simulink model "SimpleEKF_2007a"  (Simulink 6.6)
settings: Solver=FixedStepDiscrete  StartTime=0.0  StopTime=300  FixedStep=0.01  RelTol=1e-3
values from neighbouring files (symbols this model uses):
  initP = diag([ 1 1 1 1e5 1e5 1 1e5 1e5 1e5 ])    [SimpleEKF_init.m.m]
undefined symbols (not defined in the file or in its folder): DiscIntNeverNeededParam, gcbh, hwbcalib_subsystem
libraries: simulink x8, dspmtrx3 x5, dspinverses x1
(part 7 of 9)

== system SimpleEKF_2007a/INS/Attitude update/Stage1/Subsystem1/a4 ==
  attInitCon : Inport  OutDataType=fixdt(1,16,0)  OutScaling=[]
  Demux : Demux  Outputs=3
  Gain : Gain  Gain=0.5  ParameterDataType=fixdt(1,16,0)  ParameterScaling=[]  OutDataType=fixdt(1,16,0)  OutScaling=[]  SampleTime=0.01
  Gain1 : Gain  Gain=0.5  ParameterDataType=fixdt(1,16,0)  ParameterScaling=[]  OutDataType=fixdt(1,16,0)  OutScaling=[]  SampleTime=0.01
  Gain2 : Gain  Gain=0.5  ParameterDataType=fixdt(1,16,0)  ParameterScaling=[]  OutDataType=fixdt(1,16,0)  OutScaling=[]  SampleTime=0.01
  Product : Product  Inputs=3  OutDataType=fixdt(1,16,0)  OutScaling=[]  SampleTime=0.01  RndMeth=Zero
  Product1 : Product  Inputs=3  OutDataType=fixdt(1,16,0)  OutScaling=[]  SampleTime=0.01  RndMeth=Zero
  Sum : Sum  Inputs=|+-  OutDataType=fixdt(1,16,0)  OutScaling=[]  SampleTime=0.01
  Trigonometric Function : Trigonometry  Operator=cos  SampleTime=0.01
  Trigonometric Function1 : Trigonometry  Operator=cos  SampleTime=0.01
  Trigonometric Function2 : Trigonometry  SampleTime=0.01
  Trigonometric Function3 : Trigonometry
  Trigonometric Function4 : Trigonometry  Operator=cos  SampleTime=0.01
  Trigonometric Function5 : Trigonometry  SampleTime=0.01
  a2 : Outport  OutDataType=fixdt(1,16,0)  OutScaling=[]
  wires:
  attInitCon/1 -> Demux/1
  Demux/1 -> Gain2/1
  Demux/2 -> Gain/1
  Demux/3 -> Gain1/1
  Gain2/1 -> Trigonometric Function/1, Trigonometric Function3/1
  Gain/1 -> Trigonometric Function1/1, Trigonometric Function5/1
  Gain1/1 -> Trigonometric Function2/1, Trigonometric Function4/1
  Trigonometric Function/1 -> Product/1
  Trigonometric Function1/1 -> Product/2
  Trigonometric Function2/1 -> Product/3
  Product/1 -> Sum/1
  Sum/1 -> a2/1
  Product1/1 -> Sum/2
  Trigonometric Function3/1 -> Product1/1
  Trigonometric Function4/1 -> Product1/2
  Trigonometric Function5/1 -> Product1/3

== system SimpleEKF_2007a/INS/Attitude update/Stage2/Subsystem/Subsystem ==
  M11 : Inport  OutDataType=fixdt(1,16,0)  OutScaling=[]
  M21 : Inport  Port=2  OutDataType=fixdt(1,16,0)  OutScaling=[]
  M31 : Inport  Port=3  OutDataType=fixdt(1,16,0)  OutScaling=[]
  M12 : Inport  Port=4  OutDataType=fixdt(1,16,0)  OutScaling=[]
  M22 : Inport  Port=5  OutDataType=fixdt(1,16,0)  OutScaling=[]
  M32 : Inport  Port=6  OutDataType=fixdt(1,16,0)  OutScaling=[]
  M13 : Inport  Port=7  OutDataType=fixdt(1,16,0)  OutScaling=[]
  M23 : Inport  Port=8  OutDataType=fixdt(1,16,0)  OutScaling=[]
  M33 : Inport  Port=9  OutDataType=fixdt(1,16,0)  OutScaling=[]
  Mux : Mux  Inputs=9
  Reshape (9) to [3x3] column-major : Reshape  OutputDimensionality=Customize  OutputDimensions=[3,3]
  Matrix : Outport  OutDataType=fixdt(1,16,0)  OutScaling=[]
  wires:
  M33/1 -> Mux/9
  M23/1 -> Mux/8
  M13/1 -> Mux/7
  M32/1 -> Mux/6
  Reshape (9) to [3x3] column-major/1 -> Matrix/1
  M22/1 -> Mux/5
  M12/1 -> Mux/4
  M31/1 -> Mux/3
  M21/1 -> Mux/2
  M11/1 -> Mux/1
  Mux/1 -> Reshape (9) to [3x3] column-major/1

== system SimpleEKF_2007a/INS/Attitude update/Stage2/Subsystem/a11 ==
  quat : Inport  OutDataType=fixdt(1,16,0)  OutScaling=[]  Interpolate=off  mask(Inport (HW)){maskPort=1, PortWidth=0, BusOuputAsStruct=0, signalName=<, Unit=, lowerRange=, upperRange=, InitOut=, latch=Latched}
      mask prompts: maskPort "Mask Port"; PortWidth "Dimensions (-1 for dynamic):"; BusOuputAsStruct "Output as Non-Virtual:"; signalName "Signal Name"; lowerRange "Lower Range"; upperRange "Upper Range"; InitOut "Software Initial Output"; latch "DEOS Consumed Type"
      mask init:
      | %hwbcalib_inport(gcbh,'done');
      settings: CopyFcn=hwbcalib_copyfcn(gcbh);  UndoDeleteFcn=hwbcalib_inport(gcbh,'undodelete');  ModelCloseFcn=set_param(gcbh,'DeleteFcn','');  OpenFcn=hwbcalib_inport(gcbh,0);  PreDeleteFcn=hwbcalib_inport(gcbh,'delete');
      mask Help: file:///../../../Inport.html
      mask StyleString: edit,edit,edit,edit,edit,edit,edit,edit,popup(Latched|Not Latched)
      mask Display:
      | text(4,8,['quat   [' maskPort ']'],'Horizontal','left','Vertical','middle')
      | plot([0 50-10],[0 0]);
      | plot([0 0],[0 16]);
      | plot([0 50-10],[16 16]);
      | plot([50-10 50],[16 8]);
      | plot([50-10 50],[0 8]);
  BorderBottom : Subsystem
      settings: AttributesFormatString="* HONEYWELL PROPRIETARY AND CONFIDENTIAL * Copyright (c) 1996-2011 Honeywell International Inc. * Unpublished Work.  All rights reserved. *"
      mask Type: Border (HW)
      mask Description: Border
  BorderLeft : Subsystem
      mask Type: Border (HW)
      mask Description: Border
  BorderRight : Subsystem
      mask Type: Border (HW)
      mask Description: Border
  BorderTop : Subsystem
      mask Type: Border (HW)
      mask Description: Border
  Subsystem Revision : Subsystem  mask(Subsystem Revision (HW)){trace=}
      mask prompts: trace "Trace Tag:"
      settings: CopyFcn=hwbcalib_copyfcn(gcbh);  OpenFcn=hwbcalib_subrevision(gcbh,0);
      mask Help: file:///../../../Subsystem_Revision.html
      mask Display: disp('Program: \nCPU/Process: /D:\nDLL: tgen\nFilename: INS_ham_napokusy.mdl\nSubsystem: INS/Attitude update/Stage1/quatToDcm/a11\n\nHAM Library Version: 6.5.0\nRevision: -\nDate: 07-Dec-2011 at 09:52:57\nModel Update Rate: 100 Hz\n[ode3]\nTrace Tag: \n\nPage: 13 of 53, Parent Page: 12')
  deMux : Subsystem  mask(Demux (HW)){num=4}
      mask prompts: num "Number of Outputs"
      mask init:
      | %hwbcalib_doDoneCallback('hwbcalib_demux',gcbh,99);
      settings: CopyFcn=hwbcalib_copyfcn(gcbh);  OpenFcn=hwbcalib_demux(gcbh,0);
      mask Help: file:///../../../De-Multiplexer.html
  product : Subsystem  mask(Product (HW)){num=2}
      mask prompts: num "Numer of Inputs"
      mask init:
      | %hwbcalib_doDoneCallback('hwbcalib_product',gcbh,99);
      settings: CopyFcn=hwbcalib_copyfcn(gcbh);  OpenFcn=hwbcalib_product(gcbh,0);
      mask Help: file:///../../../Product.html
      mask Display: disp('X')
  product1 : Subsystem  mask(Product (HW)){num=2}
      mask prompts: num "Numer of Inputs"
      mask init:
      | %hwbcalib_doDoneCallback('hwbcalib_product',gcbh,99);
      settings: CopyFcn=hwbcalib_copyfcn(gcbh);  OpenFcn=hwbcalib_product(gcbh,0);
      mask Help: file:///../../../Product.html
      mask Display: disp('X')
  product2 : Subsystem  mask(Product (HW)){num=2}
      mask prompts: num "Numer of Inputs"
      mask init:
      | %hwbcalib_doDoneCallback('hwbcalib_product',gcbh,99);
      settings: CopyFcn=hwbcalib_copyfcn(gcbh);  OpenFcn=hwbcalib_product(gcbh,0);
      mask Help: file:///../../../Product.html
      mask Display: disp('X')
  product3 : Subsystem  mask(Product (HW)){num=2}
      mask prompts: num "Numer of Inputs"
      mask init:
      | %hwbcalib_doDoneCallback('hwbcalib_product',gcbh,99);
      settings: CopyFcn=hwbcalib_copyfcn(gcbh);  OpenFcn=hwbcalib_product(gcbh,0);
      mask Help: file:///../../../Product.html
      mask Display: disp('X')
  sum : Subsystem  mask(Sum (HW)){signs=++--}
      mask prompts: signs "String of Signs"
      mask init:
      | %hwbcalib_doDoneCallback('hwbcalib_sum',gcbh,99);
      settings: CopyFcn=hwbcalib_copyfcn(gcbh);  OpenFcn=hwbcalib_sum(gcbh,0);
      mask Help: file:///../../../Summation.html
      mask Display:
      | text(0.2, (20*(4-1)+11)/80, '+');
      | text(0.2, (20*(3-1)+11)/80, '+');
      | text(0.2, (20*(2-1)+11)/80, '-');
      | text(0.2, (20*(1-1)+11)/80, '-');
  a11 : Outport  OutDataType=fixdt(1,16,0)  OutScaling=[]  mask(Outport (HW)){maskPort=1, PortWidth=0, lowerRange=, upperRange=, signalName=<, Unit=}
      mask prompts: maskPort "Mask Port"; PortWidth "Dimensions (-1 for dynamic):"; lowerRange "Lower Range"; upperRange "Upper Range"; signalName "Signal Name"; Unit "Units"
      mask init:
      | %hwbcalib_outport(gcbh,'done');
      settings: CopyFcn=hwbcalib_copyfcn(gcbh);  UndoDeleteFcn=hwbcalib_outport(gcbh,'undodelete');  ModelCloseFcn=set_param(gcbh,'DeleteFcn','');  OpenFcn=hwbcalib_outport(gcbh,0);  PreDeleteFcn=hwbcalib_outport(gcbh,'delete');
      mask Help: file:///../../../Outport.html
      mask Display:
      | text(50-4,8,['a11   [' maskPort ']'],'Horizontal','right','Vertical','middle')
      | plot([10 50],[0 0]);
      | plot([50-1 50-1],[0 16]);
      | plot([10 50],[16 16]);
      | plot([0 10],[8 16]);
      | plot([0 10],[8 0]);
  wires:
  quat/1 -> deMux/1(Dmx)
  sum/1(1000) -> a11/1
  deMux/1(1) -> product/2(2), product/1(1)
  deMux/2(2) -> product1/1(1), product1/2(2)
  deMux/3(3) -> product2/1(1), product2/2(2)
  deMux/4(4) -> product3/2(2), product3/1(1)
  product/1(1000) -> sum/1(1)
  product1/1(1000) -> sum/2(2)
  product2/1(1000) -> sum/3(3)
  product3/1(1000) -> sum/4(4)

== system SimpleEKF_2007a/INS/Attitude update/Stage2/Subsystem/a12 ==
  quat : Inport  OutDataType=fixdt(1,16,0)  OutScaling=[]  Interpolate=off  mask(Inport (HW)){maskPort=1, PortWidth=0, BusOuputAsStruct=0, signalName=<, Unit=, lowerRange=, upperRange=, InitOut=, latch=Latched}
      mask prompts: maskPort "Mask Port"; PortWidth "Dimensions (-1 for dynamic):"; BusOuputAsStruct "Output as Non-Virtual:"; signalName "Signal Name"; lowerRange "Lower Range"; upperRange "Upper Range"; InitOut "Software Initial Output"; latch "DEOS Consumed Type"
      mask init:
      | %hwbcalib_inport(gcbh,'done');
      settings: CopyFcn=hwbcalib_copyfcn(gcbh);  UndoDeleteFcn=hwbcalib_inport(gcbh,'undodelete');  ModelCloseFcn=set_param(gcbh,'DeleteFcn','');  OpenFcn=hwbcalib_inport(gcbh,0);  PreDeleteFcn=hwbcalib_inport(gcbh,'delete');
      mask Help: file:///../../../Inport.html
      mask StyleString: edit,edit,edit,edit,edit,edit,edit,edit,popup(Latched|Not Latched)
      mask Display:
      | text(4,8,['quat   [' maskPort ']'],'Horizontal','left','Vertical','middle')
      | plot([0 50-10],[0 0]);
      | plot([0 0],[0 16]);
      | plot([0 50-10],[16 16]);
      | plot([50-10 50],[16 8]);
      | plot([50-10 50],[0 8]);
  BorderBottom : Subsystem
      settings: AttributesFormatString="* HONEYWELL PROPRIETARY AND CONFIDENTIAL * Copyright (c) 1996-2011 Honeywell International Inc. * Unpublished Work.  All rights reserved. *"
      mask Type: Border (HW)
      mask Description: Border
  BorderLeft : Subsystem
      mask Type: Border (HW)
      mask Description: Border
  BorderRight : Subsystem
      mask Type: Border (HW)
      mask Description: Border
  BorderTop : Subsystem
      mask Type: Border (HW)
      mask Description: Border
  Subsystem Revision : Subsystem  mask(Subsystem Revision (HW)){trace=}
      mask prompts: trace "Trace Tag:"
      settings: CopyFcn=hwbcalib_copyfcn(gcbh);  OpenFcn=hwbcalib_subrevision(gcbh,0);
      mask Help: file:///../../../Subsystem_Revision.html
      mask Display: disp('Program: \nCPU/Process: /D:\nDLL: tgen\nFilename: INS_ham_napokusy.mdl\nSubsystem: INS/Attitude update/Stage1/quatToDcm/a12\n\nHAM Library Version: 6.5.0\nRevision: -\nDate: 07-Dec-2011 at 09:52:57\nModel Update Rate: 100 Hz\n[ode3]\nTrace Tag: \n\nPage: 14 of 53, Parent Page: 12')
  deMux : Subsystem  mask(Demux (HW)){num=4}
      mask prompts: num "Number of Outputs"
      mask init:
      | %hwbcalib_doDoneCallback('hwbcalib_demux',gcbh,99);
      settings: CopyFcn=hwbcalib_copyfcn(gcbh);  OpenFcn=hwbcalib_demux(gcbh,0);
      mask Help: file:///../../../De-Multiplexer.html
  gain : Subsystem  mask(Gain (HW)){gain=2, Ts=1/100}
      mask prompts: Ts "Sample Time"
      mask init:
      | %hwbcalib_doDoneCallback('hwbcalib_gain',gcbh,99);
      settings: CopyFcn=hwbcalib_copyfcn(gcbh);  OpenFcn=hwbcalib_gain(gcbh,0);
      mask Help: file:///../../../Gain.html
      mask Display: disp('k=2')
  product : Subsystem  mask(Product (HW)){num=2}
      mask prompts: num "Numer of Inputs"
      mask init:
      | %hwbcalib_doDoneCallback('hwbcalib_product',gcbh,99);
      settings: CopyFcn=hwbcalib_copyfcn(gcbh);  OpenFcn=hwbcalib_product(gcbh,0);
      mask Help: file:///../../../Product.html
      mask Display: disp('X')
  product1 : Subsystem  mask(Product (HW)){num=2}
      mask prompts: num "Numer of Inputs"
      mask init:
      | %hwbcalib_doDoneCallback('hwbcalib_product',gcbh,99);
      settings: CopyFcn=hwbcalib_copyfcn(gcbh);  OpenFcn=hwbcalib_product(gcbh,0);
      mask Help: file:///../../../Product.html
      mask Display: disp('X')
  sum : Subsystem  mask(Sum (HW)){signs=++}
      mask prompts: signs "String of Signs"
      mask init:
      | %hwbcalib_doDoneCallback('hwbcalib_sum',gcbh,99);
      settings: CopyFcn=hwbcalib_copyfcn(gcbh);  OpenFcn=hwbcalib_sum(gcbh,0);
      mask Help: file:///../../../Summation.html
      mask Display:
      | text(0.2, (20*(2-1)+11)/40, '+');
      | text(0.2, (20*(1-1)+11)/40, '+');
  a12 : Outport  OutDataType=fixdt(1,16,0)  OutScaling=[]  mask(Outport (HW)){maskPort=1, PortWidth=0, lowerRange=, upperRange=, signalName=<, Unit=}
      mask prompts: maskPort "Mask Port"; PortWidth "Dimensions (-1 for dynamic):"; lowerRange "Lower Range"; upperRange "Upper Range"; signalName "Signal Name"; Unit "Units"
      mask init:
      | %hwbcalib_outport(gcbh,'done');
      settings: CopyFcn=hwbcalib_copyfcn(gcbh);  UndoDeleteFcn=hwbcalib_outport(gcbh,'undodelete');  ModelCloseFcn=set_param(gcbh,'DeleteFcn','');  OpenFcn=hwbcalib_outport(gcbh,0);  PreDeleteFcn=hwbcalib_outport(gcbh,'delete');
      mask Help: file:///../../../Outport.html
      mask Display:
      | text(50-4,8,['a12   [' maskPort ']'],'Horizontal','right','Vertical','middle')
      | plot([10 50],[0 0]);
      | plot([50-1 50-1],[0 16]);
      | plot([10 50],[16 16]);
      | plot([0 10],[8 16]);
      | plot([0 10],[8 0]);
  wires:
  quat/1 -> deMux/1(Dmx)
  deMux/1(1) -> product/2(2)
  deMux/4(4) -> product/1(1)
  product/1(1000) -> sum/1(1)
  product1/1(1000) -> sum/2(2)
  deMux/2(2) -> product1/1(1)
  deMux/3(3) -> product1/2(2)
  sum/1(1000) -> gain/1(1)
  gain/1(2) -> a12/1

== system SimpleEKF_2007a/INS/Attitude update/Stage2/Subsystem/a13 ==
  quat : Inport  OutDataType=fixdt(1,16,0)  OutScaling=[]  Interpolate=off  mask(Inport (HW)){maskPort=1, PortWidth=0, BusOuputAsStruct=0, signalName=<, Unit=, lowerRange=, upperRange=, InitOut=, latch=Latched}
      mask prompts: maskPort "Mask Port"; PortWidth "Dimensions (-1 for dynamic):"; BusOuputAsStruct "Output as Non-Virtual:"; signalName "Signal Name"; lowerRange "Lower Range"; upperRange "Upper Range"; InitOut "Software Initial Output"; latch "DEOS Consumed Type"
      mask init:
      | %hwbcalib_inport(gcbh,'done');
      settings: CopyFcn=hwbcalib_copyfcn(gcbh);  UndoDeleteFcn=hwbcalib_inport(gcbh,'undodelete');  ModelCloseFcn=set_param(gcbh,'DeleteFcn','');  OpenFcn=hwbcalib_inport(gcbh,0);  PreDeleteFcn=hwbcalib_inport(gcbh,'delete');
      mask Help: file:///../../../Inport.html
      mask StyleString: edit,edit,edit,edit,edit,edit,edit,edit,popup(Latched|Not Latched)
      mask Display:
      | text(4,8,['quat   [' maskPort ']'],'Horizontal','left','Vertical','middle')
      | plot([0 50-10],[0 0]);
      | plot([0 0],[0 16]);
      | plot([0 50-10],[16 16]);
      | plot([50-10 50],[16 8]);
      | plot([50-10 50],[0 8]);
  BorderBottom : Subsystem
      settings: AttributesFormatString="* HONEYWELL PROPRIETARY AND CONFIDENTIAL * Copyright (c) 1996-2011 Honeywell International Inc. * Unpublished Work.  All rights reserved. *"
      mask Type: Border (HW)
      mask Description: Border
  BorderLeft : Subsystem
      mask Type: Border (HW)
      mask Description: Border
  BorderRight : Subsystem
      mask Type: Border (HW)
      mask Description: Border
  BorderTop : Subsystem
      mask Type: Border (HW)
      mask Description: Border
  Subsystem Revision : Subsystem  mask(Subsystem Revision (HW)){trace=}
      mask prompts: trace "Trace Tag:"
      settings: CopyFcn=hwbcalib_copyfcn(gcbh);  OpenFcn=hwbcalib_subrevision(gcbh,0);
      mask Help: file:///../../../Subsystem_Revision.html
      mask Display: disp('Program: \nCPU/Process: /D:\nDLL: tgen\nFilename: INS_ham_napokusy.mdl\nSubsystem: INS/Attitude update/Stage1/quatToDcm/a13\n\nHAM Library Version: 6.5.0\nRevision: -\nDate: 07-Dec-2011 at 09:52:57\nModel Update Rate: 100 Hz\n[ode3]\nTrace Tag: \n\nPage: 15 of 53, Parent Page: 12')
  deMux : Subsystem  mask(Demux (HW)){num=4}
      mask prompts: num "Number of Outputs"
      mask init:
      | %hwbcalib_doDoneCallback('hwbcalib_demux',gcbh,99);
      settings: CopyFcn=hwbcalib_copyfcn(gcbh);  OpenFcn=hwbcalib_demux(gcbh,0);
      mask Help: file:///../../../De-Multiplexer.html
  gain : Subsystem  mask(Gain (HW)){gain=2, Ts=1/100}
      mask prompts: Ts "Sample Time"
      mask init:
      | %hwbcalib_doDoneCallback('hwbcalib_gain',gcbh,99);
      settings: CopyFcn=hwbcalib_copyfcn(gcbh);  OpenFcn=hwbcalib_gain(gcbh,0);
      mask Help: file:///../../../Gain.html
      mask Display: disp('k=2')
  product : Subsystem  mask(Product (HW)){num=2}
      mask prompts: num "Numer of Inputs"
      mask init:
      | %hwbcalib_doDoneCallback('hwbcalib_product',gcbh,99);
      settings: CopyFcn=hwbcalib_copyfcn(gcbh);  OpenFcn=hwbcalib_product(gcbh,0);
      mask Help: file:///../../../Product.html
      mask Display: disp('X')
  product1 : Subsystem  mask(Product (HW)){num=2}
      mask prompts: num "Numer of Inputs"
      mask init:
      | %hwbcalib_doDoneCallback('hwbcalib_product',gcbh,99);
      settings: CopyFcn=hwbcalib_copyfcn(gcbh);  OpenFcn=hwbcalib_product(gcbh,0);
      mask Help: file:///../../../Product.html
      mask Display: disp('X')
  sum : Subsystem  mask(Sum (HW)){signs=-+}
      mask prompts: signs "String of Signs"
      mask init:
      | %hwbcalib_doDoneCallback('hwbcalib_sum',gcbh,99);
      settings: CopyFcn=hwbcalib_copyfcn(gcbh);  OpenFcn=hwbcalib_sum(gcbh,0);
      mask Help: file:///../../../Summation.html
      mask Display:
      | text(0.2, (20*(2-1)+11)/40, '-');
      | text(0.2, (20*(1-1)+11)/40, '+');
  a13 : Outport  OutDataType=fixdt(1,16,0)  OutScaling=[]  mask(Outport (HW)){maskPort=1, PortWidth=0, lowerRange=, upperRange=, signalName=<, Unit=}
      mask prompts: maskPort "Mask Port"; PortWidth "Dimensions (-1 for dynamic):"; lowerRange "Lower Range"; upperRange "Upper Range"; signalName "Signal Name"; Unit "Units"
      mask init:
      | %hwbcalib_outport(gcbh,'done');
      settings: CopyFcn=hwbcalib_copyfcn(gcbh);  UndoDeleteFcn=hwbcalib_outport(gcbh,'undodelete');  ModelCloseFcn=set_param(gcbh,'DeleteFcn','');  OpenFcn=hwbcalib_outport(gcbh,0);  PreDeleteFcn=hwbcalib_outport(gcbh,'delete');
      mask Help: file:///../../../Outport.html
      mask Display:
      | text(50-4,8,['a13   [' maskPort ']'],'Horizontal','right','Vertical','middle')
      | plot([10 50],[0 0]);
      | plot([50-1 50-1],[0 16]);
      | plot([10 50],[16 16]);
      | plot([0 10],[8 16]);
      | plot([0 10],[8 0]);
  wires:
  quat/1 -> deMux/1(Dmx)
  product/1(1000) -> sum/1(1)
  product1/1(1000) -> sum/2(2)
  sum/1(1000) -> gain/1(1)
  gain/1(2) -> a13/1
  deMux/1(1) -> product/1(1)
  deMux/3(3) -> product/2(2)
  deMux/2(2) -> product1/1(1)
  deMux/4(4) -> product1/2(2)

== system SimpleEKF_2007a/INS/Attitude update/Stage2/Subsystem/a21 ==
  quat : Inport  OutDataType=fixdt(1,16,0)  OutScaling=[]  Interpolate=off  mask(Inport (HW)){maskPort=1, PortWidth=0, BusOuputAsStruct=0, signalName=<, Unit=, lowerRange=, upperRange=, InitOut=, latch=Latched}
      mask prompts: maskPort "Mask Port"; PortWidth "Dimensions (-1 for dynamic):"; BusOuputAsStruct "Output as Non-Virtual:"; signalName "Signal Name"; lowerRange "Lower Range"; upperRange "Upper Range"; InitOut "Software Initial Output"; latch "DEOS Consumed Type"
      mask init:
      | %hwbcalib_inport(gcbh,'done');
      settings: CopyFcn=hwbcalib_copyfcn(gcbh);  UndoDeleteFcn=hwbcalib_inport(gcbh,'undodelete');  ModelCloseFcn=set_param(gcbh,'DeleteFcn','');  OpenFcn=hwbcalib_inport(gcbh,0);  PreDeleteFcn=hwbcalib_inport(gcbh,'delete');
      mask Help: file:///../../../Inport.html
      mask StyleString: edit,edit,edit,edit,edit,edit,edit,edit,popup(Latched|Not Latched)
      mask Display:
      | text(4,8,['quat   [' maskPort ']'],'Horizontal','left','Vertical','middle')
      | plot([0 50-10],[0 0]);
      | plot([0 0],[0 16]);
      | plot([0 50-10],[16 16]);
      | plot([50-10 50],[16 8]);
      | plot([50-10 50],[0 8]);
  BorderBottom : Subsystem
      settings: AttributesFormatString="* HONEYWELL PROPRIETARY AND CONFIDENTIAL * Copyright (c) 1996-2011 Honeywell International Inc. * Unpublished Work.  All rights reserved. *"
      mask Type: Border (HW)
      mask Description: Border
  BorderLeft : Subsystem
      mask Type: Border (HW)
      mask Description: Border
  BorderRight : Subsystem
      mask Type: Border (HW)
      mask Description: Border
  BorderTop : Subsystem
      mask Type: Border (HW)
      mask Description: Border
  Subsystem Revision : Subsystem  mask(Subsystem Revision (HW)){trace=}
      mask prompts: trace "Trace Tag:"
      settings: CopyFcn=hwbcalib_copyfcn(gcbh);  OpenFcn=hwbcalib_subrevision(gcbh,0);
      mask Help: file:///../../../Subsystem_Revision.html
      mask Display: disp('Program: \nCPU/Process: /D:\nDLL: tgen\nFilename: INS_ham_napokusy.mdl\nSubsystem: INS/Attitude update/Stage1/quatToDcm/a21\n\nHAM Library Version: 6.5.0\nRevision: -\nDate: 07-Dec-2011 at 09:52:57\nModel Update Rate: 100 Hz\n[ode3]\nTrace Tag: \n\nPage: 16 of 53, Parent Page: 12')
  deMux : Subsystem  mask(Demux (HW)){num=4}
      mask prompts: num "Number of Outputs"
      mask init:
      | %hwbcalib_doDoneCallback('hwbcalib_demux',gcbh,99);
      settings: CopyFcn=hwbcalib_copyfcn(gcbh);  OpenFcn=hwbcalib_demux(gcbh,0);
      mask Help: file:///../../../De-Multiplexer.html
  gain : Subsystem  mask(Gain (HW)){gain=2, Ts=1/100}
      mask prompts: Ts "Sample Time"
      mask init:
      | %hwbcalib_doDoneCallback('hwbcalib_gain',gcbh,99);
      settings: CopyFcn=hwbcalib_copyfcn(gcbh);  OpenFcn=hwbcalib_gain(gcbh,0);
      mask Help: file:///../../../Gain.html
      mask Display: disp('k=2')
  product : Subsystem  mask(Product (HW)){num=2}
      mask prompts: num "Numer of Inputs"
      mask init:
      | %hwbcalib_doDoneCallback('hwbcalib_product',gcbh,99);
      settings: CopyFcn=hwbcalib_copyfcn(gcbh);  OpenFcn=hwbcalib_product(gcbh,0);
      mask Help: file:///../../../Product.html
      mask Display: disp('X')
  product1 : Subsystem  mask(Product (HW)){num=2}
      mask prompts: num "Numer of Inputs"
      mask init:
      | %hwbcalib_doDoneCallback('hwbcalib_product',gcbh,99);
      settings: CopyFcn=hwbcalib_copyfcn(gcbh);  OpenFcn=hwbcalib_product(gcbh,0);
      mask Help: file:///../../../Product.html
      mask Display: disp('X')
  sum : Subsystem  mask(Sum (HW)){signs=-+}
      mask prompts: signs "String of Signs"
      mask init:
      | %hwbcalib_doDoneCallback('hwbcalib_sum',gcbh,99);
      settings: CopyFcn=hwbcalib_copyfcn(gcbh);  OpenFcn=hwbcalib_sum(gcbh,0);
      mask Help: file:///../../../Summation.html
      mask Display:
      | text(0.2, (20*(2-1)+11)/40, '-');
      | text(0.2, (20*(1-1)+11)/40, '+');
  a21 : Outport  OutDataType=fixdt(1,16,0)  OutScaling=[]  mask(Outport (HW)){maskPort=1, PortWidth=0, lowerRange=, upperRange=, signalName=<, Unit=}
      mask prompts: maskPort "Mask Port"; PortWidth "Dimensions (-1 for dynamic):"; lowerRange "Lower Range"; upperRange "Upper Range"; signalName "Signal Name"; Unit "Units"
      mask init:
      | %hwbcalib_outport(gcbh,'done');
      settings: CopyFcn=hwbcalib_copyfcn(gcbh);  UndoDeleteFcn=hwbcalib_outport(gcbh,'undodelete');  ModelCloseFcn=set_param(gcbh,'DeleteFcn','');  OpenFcn=hwbcalib_outport(gcbh,0);  PreDeleteFcn=hwbcalib_outport(gcbh,'delete');
      mask Help: file:///../../../Outport.html
      mask Display:
      | text(50-4,8,['a21   [' maskPort ']'],'Horizontal','right','Vertical','middle')
      | plot([10 50],[0 0]);
      | plot([50-1 50-1],[0 16]);
      | plot([10 50],[16 16]);
      | plot([0 10],[8 16]);
      | plot([0 10],[8 0]);
  wires:
  quat/1 -> deMux/1(Dmx)
  deMux/1(1) -> product/2(2)
  deMux/4(4) -> product/1(1)
  product/1(1000) -> sum/1(1)
  product1/1(1000) -> sum/2(2)
  deMux/2(2) -> product1/1(1)
  deMux/3(3) -> product1/2(2)
  sum/1(1000) -> gain/1(1)
  gain/1(2) -> a21/1

== system SimpleEKF_2007a/INS/Attitude update/Stage2/Subsystem/a22 ==
  quat : Inport  OutDataType=fixdt(1,16,0)  OutScaling=[]  Interpolate=off  mask(Inport (HW)){maskPort=1, PortWidth=0, BusOuputAsStruct=0, signalName=<, Unit=, lowerRange=, upperRange=, InitOut=, latch=Latched}
      mask prompts: maskPort "Mask Port"; PortWidth "Dimensions (-1 for dynamic):"; BusOuputAsStruct "Output as Non-Virtual:"; signalName "Signal Name"; lowerRange "Lower Range"; upperRange "Upper Range"; InitOut "Software Initial Output"; latch "DEOS Consumed Type"
      mask init:
      | %hwbcalib_inport(gcbh,'done');
      settings: CopyFcn=hwbcalib_copyfcn(gcbh);  UndoDeleteFcn=hwbcalib_inport(gcbh,'undodelete');  ModelCloseFcn=set_param(gcbh,'DeleteFcn','');  OpenFcn=hwbcalib_inport(gcbh,0);  PreDeleteFcn=hwbcalib_inport(gcbh,'delete');
      mask Help: file:///../../../Inport.html
      mask StyleString: edit,edit,edit,edit,edit,edit,edit,edit,popup(Latched|Not Latched)
      mask Display:
      | text(4,8,['quat   [' maskPort ']'],'Horizontal','left','Vertical','middle')
      | plot([0 50-10],[0 0]);
      | plot([0 0],[0 16]);
      | plot([0 50-10],[16 16]);
      | plot([50-10 50],[16 8]);
      | plot([50-10 50],[0 8]);
  BorderBottom : Subsystem
      settings: AttributesFormatString="* HONEYWELL PROPRIETARY AND CONFIDENTIAL * Copyright (c) 1996-2011 Honeywell International Inc. * Unpublished Work.  All rights reserved. *"
      mask Type: Border (HW)
      mask Description: Border
  BorderLeft : Subsystem
      mask Type: Border (HW)
      mask Description: Border
  BorderRight : Subsystem
      mask Type: Border (HW)
      mask Description: Border
  BorderTop : Subsystem
      mask Type: Border (HW)
      mask Description: Border
  Subsystem Revision : Subsystem  mask(Subsystem Revision (HW)){trace=}
      mask prompts: trace "Trace Tag:"
      settings: CopyFcn=hwbcalib_copyfcn(gcbh);  OpenFcn=hwbcalib_subrevision(gcbh,0);
      mask Help: file:///../../../Subsystem_Revision.html
      mask Display: disp('Program: \nCPU/Process: /D:\nDLL: tgen\nFilename: INS_ham_napokusy.mdl\nSubsystem: INS/Attitude update/Stage1/quatToDcm/a22\n\nHAM Library Version: 6.5.0\nRevision: -\nDate: 07-Dec-2011 at 09:52:57\nModel Update Rate: 100 Hz\n[ode3]\nTrace Tag: \n\nPage: 17 of 53, Parent Page: 12')
  deMux : Subsystem  mask(Demux (HW)){num=4}
      mask prompts: num "Number of Outputs"
      mask init:
      | %hwbcalib_doDoneCallback('hwbcalib_demux',gcbh,99);
      settings: CopyFcn=hwbcalib_copyfcn(gcbh);  OpenFcn=hwbcalib_demux(gcbh,0);
      mask Help: file:///../../../De-Multiplexer.html
  product : Subsystem  mask(Product (HW)){num=2}
      mask prompts: num "Numer of Inputs"
      mask init:
      | %hwbcalib_doDoneCallback('hwbcalib_product',gcbh,99);
      settings: CopyFcn=hwbcalib_copyfcn(gcbh);  OpenFcn=hwbcalib_product(gcbh,0);
      mask Help: file:///../../../Product.html
      mask Display: disp('X')
  product1 : Subsystem  mask(Product (HW)){num=2}
      mask prompts: num "Numer of Inputs"
      mask init:
      | %hwbcalib_doDoneCallback('hwbcalib_product',gcbh,99);
      settings: CopyFcn=hwbcalib_copyfcn(gcbh);  OpenFcn=hwbcalib_product(gcbh,0);
      mask Help: file:///../../../Product.html
      mask Display: disp('X')
  product2 : Subsystem  mask(Product (HW)){num=2}
      mask prompts: num "Numer of Inputs"
      mask init:
      | %hwbcalib_doDoneCallback('hwbcalib_product',gcbh,99);
      settings: CopyFcn=hwbcalib_copyfcn(gcbh);  OpenFcn=hwbcalib_product(gcbh,0);
      mask Help: file:///../../../Product.html
      mask Display: disp('X')
  product3 : Subsystem  mask(Product (HW)){num=2}
      mask prompts: num "Numer of Inputs"
      mask init:
      | %hwbcalib_doDoneCallback('hwbcalib_product',gcbh,99);
      settings: CopyFcn=hwbcalib_copyfcn(gcbh);  OpenFcn=hwbcalib_product(gcbh,0);
      mask Help: file:///../../../Product.html
      mask Display: disp('X')
  sum : Subsystem  mask(Sum (HW)){signs=+-+-}
      mask prompts: signs "String of Signs"
      mask init:
      | %hwbcalib_doDoneCallback('hwbcalib_sum',gcbh,99);
      settings: CopyFcn=hwbcalib_copyfcn(gcbh);  OpenFcn=hwbcalib_sum(gcbh,0);
      mask Help: file:///../../../Summation.html
      mask Display:
      | text(0.2, (20*(4-1)+11)/80, '+');
      | text(0.2, (20*(3-1)+11)/80, '-');
      | text(0.2, (20*(2-1)+11)/80, '+');
      | text(0.2, (20*(1-1)+11)/80, '-');
  a22 : Outport  OutDataType=fixdt(1,16,0)  OutScaling=[]  mask(Outport (HW)){maskPort=1, PortWidth=0, lowerRange=, upperRange=, signalName=<, Unit=}
      mask prompts: maskPort "Mask Port"; PortWidth "Dimensions (-1 for dynamic):"; lowerRange "Lower Range"; upperRange "Upper Range"; signalName "Signal Name"; Unit "Units"
      mask init:
      | %hwbcalib_outport(gcbh,'done');
      settings: CopyFcn=hwbcalib_copyfcn(gcbh);  UndoDeleteFcn=hwbcalib_outport(gcbh,'undodelete');  ModelCloseFcn=set_param(gcbh,'DeleteFcn','');  OpenFcn=hwbcalib_outport(gcbh,0);  PreDeleteFcn=hwbcalib_outport(gcbh,'delete');
      mask Help: file:///../../../Outport.html
      mask Display:
      | text(50-4,8,['a22   [' maskPort ']'],'Horizontal','right','Vertical','middle')
      | plot([10 50],[0 0]);
      | plot([50-1 50-1],[0 16]);
      | plot([10 50],[16 16]);
      | plot([0 10],[8 16]);
      | plot([0 10],[8 0]);
  wires:
  quat/1 -> deMux/1(Dmx)
  sum/1(1000) -> a22/1
  deMux/1(1) -> product/2(2), product/1(1)
  deMux/2(2) -> product1/1(1), product1/2(2)
  deMux/3(3) -> product2/1(1), product2/2(2)
  deMux/4(4) -> product3/2(2), product3/1(1)
  product/1(1000) -> sum/1(1)
  product1/1(1000) -> sum/2(2)
  product2/1(1000) -> sum/3(3)
  product3/1(1000) -> sum/4(4)

== system SimpleEKF_2007a/INS/Attitude update/Stage2/Subsystem/a23 ==
  quat : Inport  OutDataType=fixdt(1,16,0)  OutScaling=[]  Interpolate=off  mask(Inport (HW)){maskPort=1, PortWidth=0, BusOuputAsStruct=0, signalName=<, Unit=, lowerRange=, upperRange=, InitOut=, latch=Latched}
      mask prompts: maskPort "Mask Port"; PortWidth "Dimensions (-1 for dynamic):"; BusOuputAsStruct "Output as Non-Virtual:"; signalName "Signal Name"; lowerRange "Lower Range"; upperRange "Upper Range"; InitOut "Software Initial Output"; latch "DEOS Consumed Type"
      mask init:
      | %hwbcalib_inport(gcbh,'done');
      settings: CopyFcn=hwbcalib_copyfcn(gcbh);  UndoDeleteFcn=hwbcalib_inport(gcbh,'undodelete');  ModelCloseFcn=set_param(gcbh,'DeleteFcn','');  OpenFcn=hwbcalib_inport(gcbh,0);  PreDeleteFcn=hwbcalib_inport(gcbh,'delete');
      mask Help: file:///../../../Inport.html
      mask StyleString: edit,edit,edit,edit,edit,edit,edit,edit,popup(Latched|Not Latched)
      mask Display:
      | text(4,8,['quat   [' maskPort ']'],'Horizontal','left','Vertical','middle')
      | plot([0 50-10],[0 0]);
      | plot([0 0],[0 16]);
      | plot([0 50-10],[16 16]);
      | plot([50-10 50],[16 8]);
      | plot([50-10 50],[0 8]);
  BorderBottom : Subsystem
      settings: AttributesFormatString="* HONEYWELL PROPRIETARY AND CONFIDENTIAL * Copyright (c) 1996-2011 Honeywell International Inc. * Unpublished Work.  All rights reserved. *"
      mask Type: Border (HW)
      mask Description: Border
  BorderLeft : Subsystem
      mask Type: Border (HW)
      mask Description: Border
  BorderRight : Subsystem
      mask Type: Border (HW)
      mask Description: Border
  BorderTop : Subsystem
      mask Type: Border (HW)
      mask Description: Border
  Subsystem Revision : Subsystem  mask(Subsystem Revision (HW)){trace=}
      mask prompts: trace "Trace Tag:"
      settings: CopyFcn=hwbcalib_copyfcn(gcbh);  OpenFcn=hwbcalib_subrevision(gcbh,0);
      mask Help: file:///../../../Subsystem_Revision.html
      mask Display: disp('Program: \nCPU/Process: /D:\nDLL: tgen\nFilename: INS_ham_napokusy.mdl\nSubsystem: INS/Attitude update/Stage1/quatToDcm/a23\n\nHAM Library Version: 6.5.0\nRevision: -\nDate: 07-Dec-2011 at 09:52:57\nModel Update Rate: 100 Hz\n[ode3]\nTrace Tag: \n\nPage: 18 of 53, Parent Page: 12')
  deMux : Subsystem  mask(Demux (HW)){num=4}
      mask prompts: num "Number of Outputs"
      mask init:
      | %hwbcalib_doDoneCallback('hwbcalib_demux',gcbh,99);
      settings: CopyFcn=hwbcalib_copyfcn(gcbh);  OpenFcn=hwbcalib_demux(gcbh,0);
      mask Help: file:///../../../De-Multiplexer.html
  gain : Subsystem  mask(Gain (HW)){gain=2, Ts=1/100}
      mask prompts: Ts "Sample Time"
      mask init:
      | %hwbcalib_doDoneCallback('hwbcalib_gain',gcbh,99);
      settings: CopyFcn=hwbcalib_copyfcn(gcbh);  OpenFcn=hwbcalib_gain(gcbh,0);
      mask Help: file:///../../../Gain.html
      mask Display: disp('k=2')
  product : Subsystem  mask(Product (HW)){num=2}
      mask prompts: num "Numer of Inputs"
      mask init:
      | %hwbcalib_doDoneCallback('hwbcalib_product',gcbh,99);
      settings: CopyFcn=hwbcalib_copyfcn(gcbh);  OpenFcn=hwbcalib_product(gcbh,0);
      mask Help: file:///../../../Product.html
      mask Display: disp('X')
  product1 : Subsystem  mask(Product (HW)){num=2}
      mask prompts: num "Numer of Inputs"
      mask init:
      | %hwbcalib_doDoneCallback('hwbcalib_product',gcbh,99);
      settings: CopyFcn=hwbcalib_copyfcn(gcbh);  OpenFcn=hwbcalib_product(gcbh,0);
      mask Help: file:///../../../Product.html
      mask Display: disp('X')
  sum : Subsystem  mask(Sum (HW)){signs=++}
      mask prompts: signs "String of Signs"
      mask init:
      | %hwbcalib_doDoneCallback('hwbcalib_sum',gcbh,99);
      settings: CopyFcn=hwbcalib_copyfcn(gcbh);  OpenFcn=hwbcalib_sum(gcbh,0);
      mask Help: file:///../../../Summation.html
      mask Display:
      | text(0.2, (20*(2-1)+11)/40, '+');
      | text(0.2, (20*(1-1)+11)/40, '+');
  a23 : Outport  OutDataType=fixdt(1,16,0)  OutScaling=[]  mask(Outport (HW)){maskPort=1, PortWidth=0, lowerRange=, upperRange=, signalName=<, Unit=}
      mask prompts: maskPort "Mask Port"; PortWidth "Dimensions (-1 for dynamic):"; lowerRange "Lower Range"; upperRange "Upper Range"; signalName "Signal Name"; Unit "Units"
      mask init:
      | %hwbcalib_outport(gcbh,'done');
      settings: CopyFcn=hwbcalib_copyfcn(gcbh);  UndoDeleteFcn=hwbcalib_outport(gcbh,'undodelete');  ModelCloseFcn=set_param(gcbh,'DeleteFcn','');  OpenFcn=hwbcalib_outport(gcbh,0);  PreDeleteFcn=hwbcalib_outport(gcbh,'delete');
      mask Help: file:///../../../Outport.html
      mask Display:
      | text(50-4,8,['a23   [' maskPort ']'],'Horizontal','right','Vertical','middle')
      | plot([10 50],[0 0]);
      | plot([50-1 50-1],[0 16]);
      | plot([10 50],[16 16]);
      | plot([0 10],[8 16]);
      | plot([0 10],[8 0]);
  wires:
  quat/1 -> deMux/1(Dmx)
  product/1(1000) -> sum/1(1)
  product1/1(1000) -> sum/2(2)
  sum/1(1000) -> gain/1(1)
  gain/1(2) -> a23/1
  deMux/1(1) -> product/1(1)
  deMux/2(2) -> product/2(2)
  deMux/3(3) -> product1/1(1)
  deMux/4(4) -> product1/2(2)

== system SimpleEKF_2007a/INS/Attitude update/Stage2/Subsystem/a31 ==
  quat : Inport  OutDataType=fixdt(1,16,0)  OutScaling=[]  Interpolate=off  mask(Inport (HW)){maskPort=1, PortWidth=0, BusOuputAsStruct=0, signalName=<, Unit=, lowerRange=, upperRange=, InitOut=, latch=Latched}
      mask prompts: maskPort "Mask Port"; PortWidth "Dimensions (-1 for dynamic):"; BusOuputAsStruct "Output as Non-Virtual:"; signalName "Signal Name"; lowerRange "Lower Range"; upperRange "Upper Range"; InitOut "Software Initial Output"; latch "DEOS Consumed Type"
      mask init:
      | %hwbcalib_inport(gcbh,'done');
      settings: CopyFcn=hwbcalib_copyfcn(gcbh);  UndoDeleteFcn=hwbcalib_inport(gcbh,'undodelete');  ModelCloseFcn=set_param(gcbh,'DeleteFcn','');  OpenFcn=hwbcalib_inport(gcbh,0);  PreDeleteFcn=hwbcalib_inport(gcbh,'delete');
      mask Help: file:///../../../Inport.html
      mask StyleString: edit,edit,edit,edit,edit,edit,edit,edit,popup(Latched|Not Latched)
      mask Display:
      | text(4,8,['quat   [' maskPort ']'],'Horizontal','left','Vertical','middle')
      | plot([0 50-10],[0 0]);
      | plot([0 0],[0 16]);
      | plot([0 50-10],[16 16]);
      | plot([50-10 50],[16 8]);
      | plot([50-10 50],[0 8]);
  BorderBottom : Subsystem
      settings: AttributesFormatString="* HONEYWELL PROPRIETARY AND CONFIDENTIAL * Copyright (c) 1996-2011 Honeywell International Inc. * Unpublished Work.  All rights reserved. *"
      mask Type: Border (HW)
      mask Description: Border
  BorderLeft : Subsystem
      mask Type: Border (HW)
      mask Description: Border
  BorderRight : Subsystem
      mask Type: Border (HW)
      mask Description: Border
  BorderTop : Subsystem
      mask Type: Border (HW)
      mask Description: Border
  Subsystem Revision : Subsystem  mask(Subsystem Revision (HW)){trace=}
      mask prompts: trace "Trace Tag:"
      settings: CopyFcn=hwbcalib_copyfcn(gcbh);  OpenFcn=hwbcalib_subrevision(gcbh,0);
      mask Help: file:///../../../Subsystem_Revision.html
      mask Display: disp('Program: \nCPU/Process: /D:\nDLL: tgen\nFilename: INS_ham_napokusy.mdl\nSubsystem: INS/Attitude update/Stage1/quatToDcm/a31\n\nHAM Library Version: 6.5.0\nRevision: -\nDate: 07-Dec-2011 at 09:52:57\nModel Update Rate: 100 Hz\n[ode3]\nTrace Tag: \n\nPage: 19 of 53, Parent Page: 12')
  deMux : Subsystem  mask(Demux (HW)){num=4}
      mask prompts: num "Number of Outputs"
      mask init:
      | %hwbcalib_doDoneCallback('hwbcalib_demux',gcbh,99);
      settings: CopyFcn=hwbcalib_copyfcn(gcbh);  OpenFcn=hwbcalib_demux(gcbh,0);
      mask Help: file:///../../../De-Multiplexer.html
  gain : Subsystem  mask(Gain (HW)){gain=2, Ts=1/100}
      mask prompts: Ts "Sample Time"
      mask init:
      | %hwbcalib_doDoneCallback('hwbcalib_gain',gcbh,99);
      settings: CopyFcn=hwbcalib_copyfcn(gcbh);  OpenFcn=hwbcalib_gain(gcbh,0);
      mask Help: file:///../../../Gain.html
      mask Display: disp('k=2')
  product : Subsystem  mask(Product (HW)){num=2}
      mask prompts: num "Numer of Inputs"
      mask init:
      | %hwbcalib_doDoneCallback('hwbcalib_product',gcbh,99);
      settings: CopyFcn=hwbcalib_copyfcn(gcbh);  OpenFcn=hwbcalib_product(gcbh,0);
      mask Help: file:///../../../Product.html
      mask Display: disp('X')
  product1 : Subsystem  mask(Product (HW)){num=2}
      mask prompts: num "Numer of Inputs"
      mask init:
      | %hwbcalib_doDoneCallback('hwbcalib_product',gcbh,99);
      settings: CopyFcn=hwbcalib_copyfcn(gcbh);  OpenFcn=hwbcalib_product(gcbh,0);
      mask Help: file:///../../../Product.html
      mask Display: disp('X')
  sum : Subsystem  mask(Sum (HW)){signs=++}
      mask prompts: signs "String of Signs"
      mask init:
      | %hwbcalib_doDoneCallback('hwbcalib_sum',gcbh,99);
      settings: CopyFcn=hwbcalib_copyfcn(gcbh);  OpenFcn=hwbcalib_sum(gcbh,0);
      mask Help: file:///../../../Summation.html
      mask Display:
      | text(0.2, (20*(2-1)+11)/40, '+');
      | text(0.2, (20*(1-1)+11)/40, '+');
  a31 : Outport  OutDataType=fixdt(1,16,0)  OutScaling=[]  mask(Outport (HW)){maskPort=1, PortWidth=0, lowerRange=, upperRange=, signalName=<, Unit=}
      mask prompts: maskPort "Mask Port"; PortWidth "Dimensions (-1 for dynamic):"; lowerRange "Lower Range"; upperRange "Upper Range"; signalName "Signal Name"; Unit "Units"
      mask init:
      | %hwbcalib_outport(gcbh,'done');
      settings: CopyFcn=hwbcalib_copyfcn(gcbh);  UndoDeleteFcn=hwbcalib_outport(gcbh,'undodelete');  ModelCloseFcn=set_param(gcbh,'DeleteFcn','');  OpenFcn=hwbcalib_outport(gcbh,0);  PreDeleteFcn=hwbcalib_outport(gcbh,'delete');
      mask Help: file:///../../../Outport.html
      mask Display:
      | text(50-4,8,['a31   [' maskPort ']'],'Horizontal','right','Vertical','middle')
      | plot([10 50],[0 0]);
      | plot([50-1 50-1],[0 16]);
      | plot([10 50],[16 16]);
      | plot([0 10],[8 16]);
      | plot([0 10],[8 0]);
  wires:
  quat/1 -> deMux/1(Dmx)
  product/1(1000) -> sum/1(1)
  product1/1(1000) -> sum/2(2)
  sum/1(1000) -> gain/1(1)
  gain/1(2) -> a31/1
  deMux/1(1) -> product/1(1)
  deMux/3(3) -> product/2(2)
  deMux/2(2) -> product1/1(1)
  deMux/4(4) -> product1/2(2)

== system SimpleEKF_2007a/INS/Attitude update/Stage2/Subsystem/a32 ==
  quat : Inport  OutDataType=fixdt(1,16,0)  OutScaling=[]  Interpolate=off  mask(Inport (HW)){maskPort=1, PortWidth=0, BusOuputAsStruct=0, signalName=<, Unit=, lowerRange=, upperRange=, InitOut=, latch=Latched}
      mask prompts: maskPort "Mask Port"; PortWidth "Dimensions (-1 for dynamic):"; BusOuputAsStruct "Output as Non-Virtual:"; signalName "Signal Name"; lowerRange "Lower Range"; upperRange "Upper Range"; InitOut "Software Initial Output"; latch "DEOS Consumed Type"
      mask init:
      | %hwbcalib_inport(gcbh,'done');
      settings: CopyFcn=hwbcalib_copyfcn(gcbh);  UndoDeleteFcn=hwbcalib_inport(gcbh,'undodelete');  ModelCloseFcn=set_param(gcbh,'DeleteFcn','');  OpenFcn=hwbcalib_inport(gcbh,0);  PreDeleteFcn=hwbcalib_inport(gcbh,'delete');
      mask Help: file:///../../../Inport.html
      mask StyleString: edit,edit,edit,edit,edit,edit,edit,edit,popup(Latched|Not Latched)
      mask Display:
      | text(4,8,['quat   [' maskPort ']'],'Horizontal','left','Vertical','middle')
      | plot([0 50-10],[0 0]);
      | plot([0 0],[0 16]);
      | plot([0 50-10],[16 16]);
      | plot([50-10 50],[16 8]);
      | plot([50-10 50],[0 8]);
  BorderBottom : Subsystem
      settings: AttributesFormatString="* HONEYWELL PROPRIETARY AND CONFIDENTIAL * Copyright (c) 1996-2011 Honeywell International Inc. * Unpublished Work.  All rights reserved. *"
      mask Type: Border (HW)
      mask Description: Border
  BorderLeft : Subsystem
      mask Type: Border (HW)
      mask Description: Border
  BorderRight : Subsystem
      mask Type: Border (HW)
      mask Description: Border
  BorderTop : Subsystem
      mask Type: Border (HW)
      mask Description: Border
  Subsystem Revision : Subsystem  mask(Subsystem Revision (HW)){trace=}
      mask prompts: trace "Trace Tag:"
      settings: CopyFcn=hwbcalib_copyfcn(gcbh);  OpenFcn=hwbcalib_subrevision(gcbh,0);
      mask Help: file:///../../../Subsystem_Revision.html
      mask Display: disp('Program: \nCPU/Process: /D:\nDLL: tgen\nFilename: INS_ham_napokusy.mdl\nSubsystem: INS/Attitude update/Stage1/quatToDcm/a32\n\nHAM Library Version: 6.5.0\nRevision: -\nDate: 07-Dec-2011 at 09:52:57\nModel Update Rate: 100 Hz\n[ode3]\nTrace Tag: \n\nPage: 20 of 53, Parent Page: 12')
  deMux : Subsystem  mask(Demux (HW)){num=4}
      mask prompts: num "Number of Outputs"
      mask init:
      | %hwbcalib_doDoneCallback('hwbcalib_demux',gcbh,99);
      settings: CopyFcn=hwbcalib_copyfcn(gcbh);  OpenFcn=hwbcalib_demux(gcbh,0);
      mask Help: file:///../../../De-Multiplexer.html
  gain : Subsystem  mask(Gain (HW)){gain=2, Ts=1/100}
      mask prompts: Ts "Sample Time"
      mask init:
      | %hwbcalib_doDoneCallback('hwbcalib_gain',gcbh,99);
      settings: CopyFcn=hwbcalib_copyfcn(gcbh);  OpenFcn=hwbcalib_gain(gcbh,0);
      mask Help: file:///../../../Gain.html
      mask Display: disp('k=2')
  product : Subsystem  mask(Product (HW)){num=2}
      mask prompts: num "Numer of Inputs"
      mask init:
      | %hwbcalib_doDoneCallback('hwbcalib_product',gcbh,99);
      settings: CopyFcn=hwbcalib_copyfcn(gcbh);  OpenFcn=hwbcalib_product(gcbh,0);
      mask Help: file:///../../../Product.html
      mask Display: disp('X')
  product1 : Subsystem  mask(Product (HW)){num=2}
      mask prompts: num "Numer of Inputs"
      mask init:
      | %hwbcalib_doDoneCallback('hwbcalib_product',gcbh,99);
      settings: CopyFcn=hwbcalib_copyfcn(gcbh);  OpenFcn=hwbcalib_product(gcbh,0);
      mask Help: file:///../../../Product.html
      mask Display: disp('X')
  sum : Subsystem  mask(Sum (HW)){signs=-+}
      mask prompts: signs "String of Signs"
      mask init:
      | %hwbcalib_doDoneCallback('hwbcalib_sum',gcbh,99);
      settings: CopyFcn=hwbcalib_copyfcn(gcbh);  OpenFcn=hwbcalib_sum(gcbh,0);
      mask Help: file:///../../../Summation.html
      mask Display:
      | text(0.2, (20*(2-1)+11)/40, '-');
      | text(0.2, (20*(1-1)+11)/40, '+');
  a32 : Outport  OutDataType=fixdt(1,16,0)  OutScaling=[]  mask(Outport (HW)){maskPort=1, PortWidth=0, lowerRange=, upperRange=, signalName=<, Unit=}
      mask prompts: maskPort "Mask Port"; PortWidth "Dimensions (-1 for dynamic):"; lowerRange "Lower Range"; upperRange "Upper Range"; signalName "Signal Name"; Unit "Units"
      mask init:
      | %hwbcalib_outport(gcbh,'done');
      settings: CopyFcn=hwbcalib_copyfcn(gcbh);  UndoDeleteFcn=hwbcalib_outport(gcbh,'undodelete');  ModelCloseFcn=set_param(gcbh,'DeleteFcn','');  OpenFcn=hwbcalib_outport(gcbh,0);  PreDeleteFcn=hwbcalib_outport(gcbh,'delete');
      mask Help: file:///../../../Outport.html
      mask Display:
      | text(50-4,8,['a32   [' maskPort ']'],'Horizontal','right','Vertical','middle')
      | plot([10 50],[0 0]);
      | plot([50-1 50-1],[0 16]);
      | plot([10 50],[16 16]);
      | plot([0 10],[8 16]);
      | plot([0 10],[8 0]);
  wires:
  quat/1 -> deMux/1(Dmx)
  product/1(1000) -> sum/1(1)
  product1/1(1000) -> sum/2(2)
  sum/1(1000) -> gain/1(1)
  gain/1(2) -> a32/1
  deMux/1(1) -> product/1(1)
  deMux/2(2) -> product/2(2)
  deMux/3(3) -> product1/1(1)
  deMux/4(4) -> product1/2(2)
